simulink model "TVModel"  (R2022a)
settings: Solver=FixedStepDiscrete  StartTime=0.0  StopTime=10.0  FixedStep=0.02  MaxStep=0.01  RelTol=1e-3
undefined symbols (not defined in the file or in its folder): MB, TV, TV_OLD
libraries: simulink x22, simulink_extras x14, slpidlib x8, fuzblock x5, controlLib x4, dspstat3 x4, eeGeneralControl x3, cstblocks x3, eeSlidingModeController x1, sharedTrackingLibrary x1
(part 1 of 8)
settings Model: Creator=giuse  LastModifiedBy=Daniele
settings SolverCC: AutoInsertRateTranBlk=on
settings OptimizationCC: DefaultParameterBehavior=Inlined  UseDivisionForNetSlopeComputation=on  GainParamInheritBuiltInType=on  UseFloatMulNetSlope=on  InlineInvariantSignals=on  PassReuseOutputArgsAs=Individual arguments  ZeroExternalMemoryAtStartup=off  ZeroInternalMemoryAtStartup=off  NoFixptDivByZeroProtection=on  EfficientFloat2IntCast=on  LifeSpan=1  OptimizeBlockOrder=speed  DifferentSizesBufferReuse=on  EfficientTunableParamExpr=on
settings DebuggingCC: ParameterTunabilityLossMsg=error  UnconnectedInputMsg=warning  UnconnectedOutputMsg=warning  UnconnectedLineMsg=warning
settings HardwareCC: ProdBitPerPointer=32  ProdBitPerSizeT=32  ProdBitPerPtrDiffT=32  ProdLargestAtomicInteger=Long  ProdLargestAtomicFloat=Double  ProdWordSize=32  ProdLongLongMode=on  ProdHWDeviceType=ARM Compatible->ARM Cortex-M
settings SFSimCC: SimCustomHeaderCode="#include \"ITB_Nucleo_configuration\\Inc\\acados_wrapper.h\""  SimUserSources=ITB_Nucleo_configuration\Src\acados_wrapper.c  MATLABDynamicMemAlloc=off  CustomCodeUndefinedFunction=DoNotDetect
settings RTWCC: SystemTargetFile=ert.tlc  GenCodeOnly=on  TemplateMakefile=ert_default_tmf  RTWUseSimCustomCode=on  CustomHeaderCode="#include \"ITB_Nucleo_configuration\\Inc\\acados_wrapper.h\""  CustomSource=ITB_Nucleo_configuration\Src\acados_wrapper.c  DLArmComputeVersion=19.05
settings CodeAppCC: ForceParamTrailComments=on  IgnoreCustomStorageClasses=off  OperatorAnnotations=on  SimulinkDataObjDesc=on  SFDataObjDesc=on  CustomSymbolStrGlobalVar=rt$N$M  CustomSymbolStrType=$N$M  CustomSymbolStrFcn=$N$M$F  CustomSymbolStrMacro=$N$M  InsertBlockDesc=on
settings ERTTargetCC: TargetLangStandard=C99 (ISO)  GenerateSampleERTMain=on  IncludeMdlTerminateFcn=off  CombineOutputUpdateFcns=off  CombineSignalStateStructs=on  SupportAbsoluteTime=off  SupportComplex=off  SupportNonInlinedSFcns=on  InlinedParameterPlacement=NonHierarchical  ERTCustomFileTemplate=example_file_process.tlc  ERTFilePackagingFormat=CompactWithDataFile

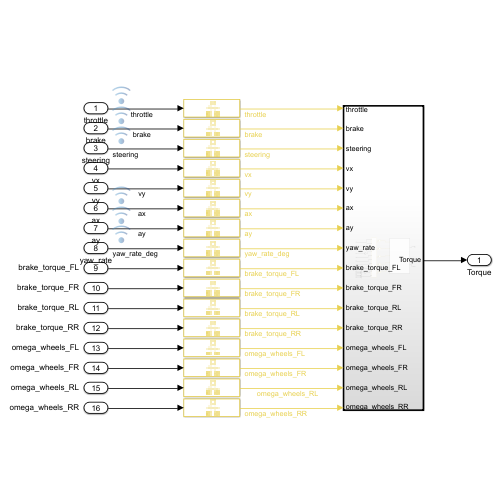
[thumbnail: Simulink's stored preview of the top-level diagram]
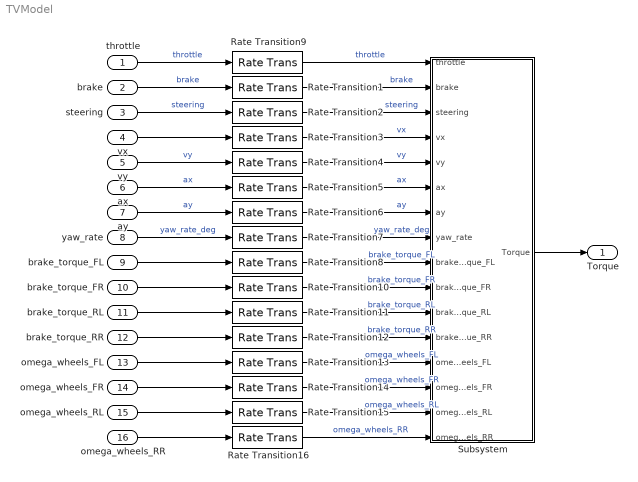
== system TVModel ==
  throttle : Inport  PortDimensions=1
  brake : Inport  Port=2  PortDimensions=1
  steering : Inport  Port=3  PortDimensions=1
  vx : Inport  Port=4  PortDimensions=1
  vy : Inport  Port=5  PortDimensions=1
  ax : Inport  Port=6  PortDimensions=1
  ay : Inport  Port=7  PortDimensions=1
  yaw_rate : Inport  Port=8  PortDimensions=1
  brake_torque_FL : Inport  Port=9  PortDimensions=1
  brake_torque_FR : Inport  Port=10  PortDimensions=1
  brake_torque_RL : Inport  Port=11  PortDimensions=1
  brake_torque_RR : Inport  Port=12  PortDimensions=1
  omega_wheels_FL : Inport  Port=13  PortDimensions=1
  omega_wheels_FR : Inport  Port=14  PortDimensions=1
  omega_wheels_RL : Inport  Port=15  PortDimensions=1
  omega_wheels_RR : Inport  Port=16  PortDimensions=1
  Rate Transition{1..16} (16 alike) : RateTransition  OutPortSampleTime=TV.MPC.T/TV.MPC.N
  Subsystem : Subsystem  TreatAsAtomicUnit=on  PartitionName=Subsystem
  Torque : Outport
  wires:
  vy/1 -> Rate Transition4/1  "vy"
  ax/1 -> Rate Transition5/1  "ax"
  brake/1 -> Rate Transition1/1  "brake"
  ay/1 -> Rate Transition6/1  "ay"
  brake_torque_RL/1 -> Rate Transition11/1
  brake_torque_RR/1 -> Rate Transition12/1
  omega_wheels_RR/1 -> Rate Transition16/1
  omega_wheels_FL/1 -> Rate Transition13/1
  brake_torque_FR/1 -> Rate Transition10/1
  yaw_rate/1 -> Rate Transition7/1  "yaw_rate_deg"
  omega_wheels_FR/1 -> Rate Transition14/1
  omega_wheels_RL/1 -> Rate Transition15/1
  steering/1 -> Rate Transition2/1  "steering"
  brake_torque_FL/1 -> Rate Transition8/1
  vx/1 -> Rate Transition3/1
  throttle/1 -> Rate Transition9/1  "throttle"
  Subsystem/1(Torque) -> Torque/1
  Rate Transition9/1 -> Subsystem/1(throttle)  "throttle"
  Rate Transition1/1 -> Subsystem/2(brake)  "brake"
  Rate Transition2/1 -> Subsystem/3(steering)  "steering"
  Rate Transition3/1 -> Subsystem/4(vx)  "vx"
  Rate Transition4/1 -> Subsystem/5(vy)  "vy"
  Rate Transition5/1 -> Subsystem/6(ax)  "ax"
  Rate Transition6/1 -> Subsystem/7(ay)  "ay"
  Rate Transition7/1 -> Subsystem/8(yaw_rate)  "yaw_rate_deg"
  Rate Transition8/1 -> Subsystem/9(brake_torque_FL)  "brake_torque_FL"
  Rate Transition10/1 -> Subsystem/10(brake_torque_FR)  "brake_torque_FR"
  Rate Transition11/1 -> Subsystem/11(brake_torque_RL)  "brake_torque_RL"
  Rate Transition12/1 -> Subsystem/12(brake_torque_RR)  "brake_torque_RR"
  Rate Transition13/1 -> Subsystem/13(omega_wheels_FL)  "omega_wheels_FL"
  Rate Transition14/1 -> Subsystem/14(omega_wheels_FR)  "omega_wheels_FR"
  Rate Transition15/1 -> Subsystem/15(omega_wheels_RL)  "omega_wheels_RL"
  Rate Transition16/1 -> Subsystem/16(omega_wheels_RR)  "omega_wheels_RR"

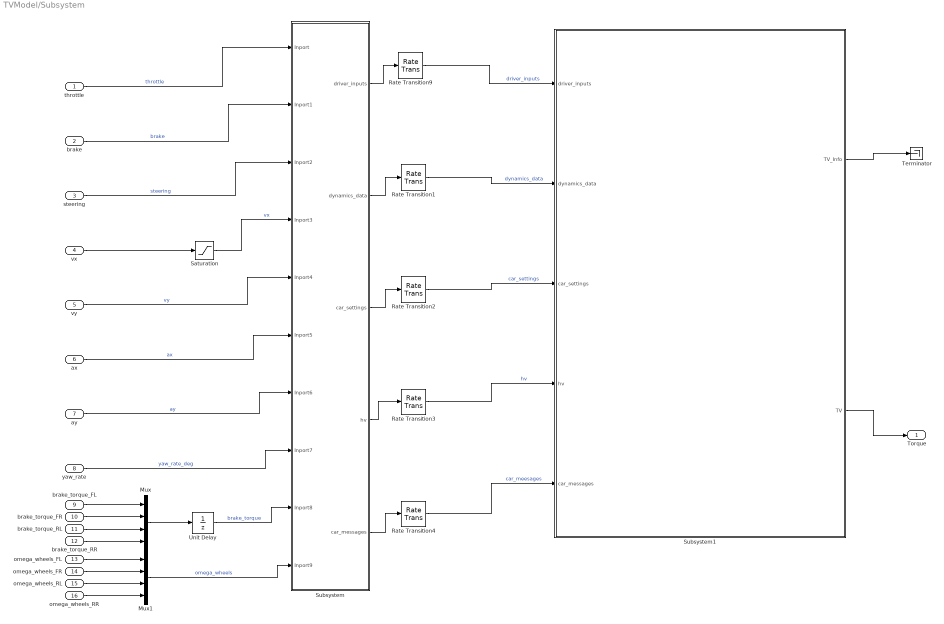
== system TVModel/Subsystem ==
  throttle : Inport  SampleTime=0.02
  brake : Inport  Port=2
  steering : Inport  Port=3
  vx : Inport  Port=4
  vy : Inport  Port=5
  ax : Inport  Port=6
  ay : Inport  Port=7
  yaw_rate : Inport  Port=8
  brake_torque_FL : Inport  Port=9
  brake_torque_FR : Inport  Port=10
  brake_torque_RL : Inport  Port=11
  brake_torque_RR : Inport  Port=12
  omega_wheels_FL : Inport  Port=13
  omega_wheels_FR : Inport  Port=14
  omega_wheels_RL : Inport  Port=15
  omega_wheels_RR : Inport  Port=16
  Mux : Mux
  Mux1 : Mux
  Rate Transition{1..4,9} (5 alike) : RateTransition  OutPortSampleTime=TV.MPC.T/TV.MPC.N
  Saturation : Saturate  UpperLimit=inf  LowerLimit=0
  Subsystem : Subsystem
  Subsystem1 : Subsystem
  Terminator : Terminator
  Unit Delay : UnitDelay  SampleTime=-1  HasFrameUpgradeWarning=on
  Torque : Outport
  wires:
  omega_wheels_FL/1 -> Mux1/1
  ax/1 -> Subsystem/6(Inport5)  "ax"
  Unit Delay/1 -> Subsystem/9(Inport8)  "brake_torque"
  vy/1 -> Subsystem/5(Inport4)  "vy"
  ay/1 -> Subsystem/7(Inport6)  "ay"
  Mux1/1 -> Subsystem/10(Inport9)  "omega_wheels"
  Saturation/1 -> Subsystem/4(Inport3)  "vx"
  brake/1 -> Subsystem/2(Inport1)  "brake"
  yaw_rate/1 -> Subsystem/8(Inport7)  "yaw_rate_deg"
  throttle/1 -> Subsystem/1(Inport)  "throttle"
  brake_torque_RL/1 -> Mux/3
  vx/1 -> Saturation/1
  brake_torque_FL/1 -> Mux/1
  omega_wheels_RR/1 -> Mux1/4
  brake_torque_RR/1 -> Mux/4
  steering/1 -> Subsystem/3(Inport2)  "steering"
  omega_wheels_FR/1 -> Mux1/2
  Mux/1 -> Unit Delay/1
  omega_wheels_RL/1 -> Mux1/3
  brake_torque_FR/1 -> Mux/2
  Subsystem/1(driver_inputs) -> Rate Transition9/1
  Subsystem/2(dynamics_data) -> Rate Transition1/1
  Subsystem/5(car_messages) -> Rate Transition4/1
  Subsystem/3(car_settings) -> Rate Transition2/1
  Rate Transition4/1 -> Subsystem1/5(car_messages)  "car_meesages"
  Rate Transition3/1 -> Subsystem1/4(hv)  "hv"
  Rate Transition2/1 -> Subsystem1/3(car_settings)  "car_settings"
  Rate Transition1/1 -> Subsystem1/2(dynamics_data)  "dynamics_data"
  Subsystem1/2(TV) -> Torque/1
  Subsystem1/1(TV_Info) -> Terminator/1
  Rate Transition9/1 -> Subsystem1/1(driver_inputs)  "driver_inputs"
  Subsystem/4(hv) -> Rate Transition3/1

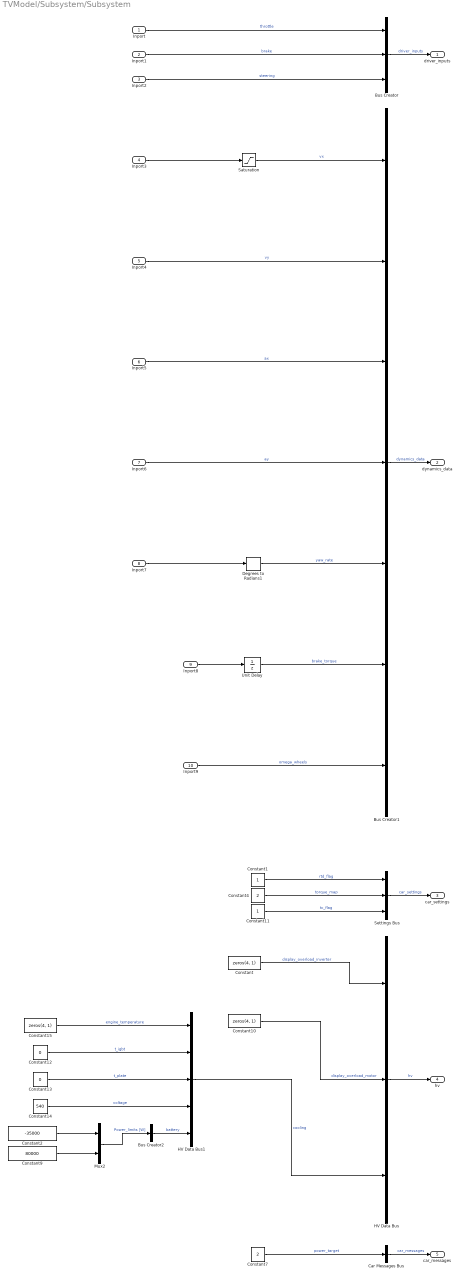
== system TVModel/Subsystem/Subsystem ==
  Inport : Inport
  Inport1 : Inport  Port=2
  Inport2 : Inport  Port=3
  Inport3 : Inport  Port=4
  Inport4 : Inport  Port=5
  Inport5 : Inport  Port=6
  Inport6 : Inport  Port=7
  Inport7 : Inport  Port=8
  Inport8 : Inport  Port=9
  Inport9 : Inport  Port=10
  Bus Creator : BusCreator  Inputs=3
  Bus Creator1 : BusCreator  Inputs=7
  Bus Creator2 : BusCreator  Inputs=1
  Car Messages Bus : BusCreator  Inputs=1
  Constant : Constant  Value=zeros(4, 1)
  Constant1 : Constant  OutDataTypeStr=uint8
  Constant10 : Constant  Value=zeros(4, 1)
  Constant11 : Constant  OutDataTypeStr=uint8
  Constant12 : Constant  Value=0
  Constant13 : Constant  Value=0
  Constant14 : Constant  Value=540
  Constant15 : Constant  Value=zeros(4, 1)
  Constant2 : Constant  Value=-35000
  Constant4 : Constant  Value=2  OutDataTypeStr=uint8
  Constant7 : Constant  Value=2
  Constant9 : Constant  Value=80000
  Degrees to Radians1 : simulink_extras/Transformations/Degrees to Radians
  HV Data Bus : BusCreator  Inputs=3
  HV Data Bus1 : BusCreator  Inputs=5
  Mux2 : Mux  Inputs=2
  Saturation : Saturate  UpperLimit=inf  LowerLimit=0
  Settings Bus : BusCreator  Inputs=3
  Unit Delay : UnitDelay  SampleTime=-1  HasFrameUpgradeWarning=on
  driver_inputs : Outport
  dynamics_data : Outport  Port=2
  car_settings : Outport  Port=3
  hv : Outport  Port=4
  car_messages : Outport  Port=5
  wires:
  Constant4/1 -> Settings Bus/2  "torque_map"
  Inport2/1 -> Bus Creator/3  "steering"
  Constant1/1 -> Settings Bus/1  "rtd_flag"
  Car Messages Bus/1 -> car_messages/1  "car_messages"
  Inport9/1 -> Bus Creator1/7  "omega_wheels"
  Degrees to Radians1/1 -> Bus Creator1/5  "yaw_rate"
  Constant7/1 -> Car Messages Bus/1  "power_target"
  Bus Creator/1 -> driver_inputs/1  "driver_inputs"
  Inport7/1 -> Degrees to Radians1/1
  Settings Bus/1 -> car_settings/1  "car_settings"
  Bus Creator1/1 -> dynamics_data/1  "dynamics_data"
  Constant11/1 -> Settings Bus/3  "tc_flag"
  Inport6/1 -> Bus Creator1/4  "ay"
  Inport5/1 -> Bus Creator1/3  "ax"
  Inport4/1 -> Bus Creator1/2  "vy"
  Inport/1 -> Bus Creator/1  "throttle"
  Unit Delay/1 -> Bus Creator1/6  "brake_torque"
  Inport8/1 -> Unit Delay/1
  Inport1/1 -> Bus Creator/2  "brake"
  Saturation/1 -> Bus Creator1/1  "vx"
  Inport3/1 -> Saturation/1
  HV Data Bus/1 -> hv/1  "hv"
  Mux2/1 -> Bus Creator2/1  "Power_limits [W]"
  Constant10/1 -> HV Data Bus/2  "display_overload_motor"
  HV Data Bus1/1 -> HV Data Bus/3  "cooling"
  Constant/1 -> HV Data Bus/1  "display_overload_inverter"
  Constant14/1 -> HV Data Bus1/4  "voltage"
  Constant12/1 -> HV Data Bus1/2  "t_igbt"
  Constant2/1 -> Mux2/1
  Constant13/1 -> HV Data Bus1/3  "t_plate"
  Constant9/1 -> Mux2/2
  Bus Creator2/1 -> HV Data Bus1/5  "battery"
  Constant15/1 -> HV Data Bus1/1  "engine_temperature"

== system TVModel/Subsystem/Subsystem1 ==
  In Bus Element2 : Inport  PortName=driver_inputs
  In Bus Element5 : Inport  PortName=driver_inputs
  In Bus Element11 : Inport  PortName=driver_inputs
  In Bus Element3 : Inport  Port=2  PortName=dynamics_data
  In Bus Element4 : Inport  Port=2  PortName=dynamics_data
  In Bus Element8 : Inport  Port=2  PortName=dynamics_data
  In Bus Element6 : Inport  Port=3  PortName=car_settings
  In Bus Element10 : Inport  Port=3  PortName=car_settings
  In Bus Element1 : Inport  Port=3  PortName=car_settings
  In Bus Element7 : Inport  Port=4  PortName=hv
  In Bus Element9 : Inport  Port=4  PortName=hv
  In Bus Element : Inport  Port=5  PortName=car_messages
  Data Store_General_Params : DataStoreMemory  DataStoreName=General_Params  WriteAfterWriteMsg=warning  WriteAfterReadMsg=warning  InitialValue=TV.LV.GENERAL  ShowAdditionalParam=off  OutDataTypeStr=Bus: zGeneral_Params
  Data Store_Map_Params : DataStoreMemory  DataStoreName=Map_Params  WriteAfterWriteMsg=warning  WriteAfterReadMsg=warning  InitialValue=TV.LV.MAP  ShowAdditionalParam=off  OutDataTypeStr=Bus: zMap_Params
  Slip Control : Subsystem
      settings: PortSchema="{\"entries\":[{\"content\":{\"sides\":[{\"content\":{\"connectorIds\":[\"In1\",\"In2\",\"In3\",\"In4\",\"In5\",\"In6\"]},\"type\":\"ConnectorPlacement.EquallySpacedRectSide\",\"uuid\":\"0a8dcb05-2d5e-427e-b3e7-e0a9c36078aa\"},{\"content\":{\"connectorIds\":[\"Out1\",\"Out2\"],\"side\":\"RIGHT\"},\"type\":\"ConnectorPlacement.EquallySpacedRectSide\",\"uuid\":\"4a483d6b-4a8b-4193-8822-91ed85f9d11c\"},{\"content\":{\"connectorIds\":[\"Out3\"],\"side\":\"TOP\"},\"type\":\"ConnectorPlacement.EquallySpacedRectSide\",\"uuid\":\"653aa866-b257-425a-9060-0af71437e8f6\"}]},\"type\":\"ConnectorPlacement.EquallySpacedConnector\",\"uuid\":\"85fc9358-bdaa-4ddd-978c-a41ea6d8fd7a\"}],\"packageUris\":[\"http://schema.mathworks.com/mf0/Connector/R2020b\"],\"version\":\"1.0\"}"
      mask Display: image('$imagefile'); % Use "Edit Image" on toolstrip to change.
  Terminator : Terminator
  Torque Distribution : Subsystem
      settings: PortSchema="{\"entries\":[{\"content\":{\"sides\":[{\"content\":{\"connectorIds\":[\"In1\",\"In2\",\"In3\",\"In4\",\"In5\",\"In6\",\"In7\",\"In8\",\"Out3\",\"In9\"]},\"type\":\"ConnectorPlacement.EquallySpacedRectSide\",\"uuid\":\"ece1a4aa-f225-4de9-8190-960458904133\"},{\"content\":{\"connectorIds\":[\"Out1\",\"Out2\"],\"side\":\"RIGHT\"},\"type\":\"ConnectorPlacement.EquallySpacedRectSide\",\"uuid\":\"588db727-2c2c-47b1-ab80-0176258858bf\"},{\"content\":{\"connectorIds\":[],\"side\":\"TOP\"},\"type\":\"ConnectorPlacement.EquallySpacedRectSide\",\"uuid\":\"54ce6245-2304-4750-b056-247655cbbdc1\"}]},\"type\":\"ConnectorPlacement.EquallySpacedConnector\",\"uuid\":\"9c8e646c-fa54-49ed-932c-87ddbb4d1884\"}],\"packageUris\":[\"http://schema.mathworks.com/mf0/Connector/R2020b\"],\"version\":\"1.0\"}"
      mask Display: image('$imagefile'); % Use "Edit Image" on toolstrip to change.
  Torque Limits : Subsystem
      mask Display: image('$imagefile'); % Use "Edit Image" on toolstrip to change.
  regen_brake : Subsystem
  steering_to_front_wheels : Subsystem
  Out Bus Element4 : Outport  PortName=TV_Info  Element=Torque_Distribution
  Out Bus Element6 : Outport  PortName=TV_Info  Element=Input_Signals.hv
  Out Bus Element7 : Outport  PortName=TV_Info  Element=Input_Signals.car_settings
  Out Bus Element8 : Outport  PortName=TV_Info  Element=Input_Signals.dynamics_data
  Out Bus Element9 : Outport  PortName=TV_Info  Element=Input_Signals.driver_inputs
  Out Bus Element10 : Outport  PortName=TV_Info  Element=Slip_Control
  Out Bus Element : Outport  Port=2  PortName=TV
  wires:
  regen_brake/1(brake_signal) -> Torque Distribution/3(brake_signal)
  In Bus Element8/1 -> Torque Limits/2(dynamics_data), Out Bus Element8/1  "dynamics_data"
  In Bus Element10/1 -> Torque Distribution/7(Car_Settings)
  In Bus Element2/1 -> steering_to_front_wheels/1(driver_inputs), regen_brake/1(driver_inputs), Torque Distribution/2(driver_inputs)
  steering_to_front_wheels/1(front_wheels_steering) -> Torque Distribution/4(front_wheels_steering), Slip Control/1(front_wheels_steering)
  In Bus Element3/1 -> Torque Distribution/1(dynamics_data)
  In Bus Element4/1 -> Slip Control/2(dynamics_data)
  Slip Control/2(slip_ratio) -> Torque Distribution/6(slip_ratio)
  Torque Distribution/1(TV_info) -> Out Bus Element4/1
  Torque Limits/1(torque_limits) -> Torque Distribution/9(torque_limits), Slip Control/4(torque_limits)
  Torque Distribution/2(TV) -> Out Bus Element/1
  Torque Distribution/3(TC_torque_out) -> Slip Control/5(tv)
  Slip Control/3(TV_Info) -> Out Bus Element10/1
  In Bus Element7/1 -> Out Bus Element6/1, Torque Limits/4(hv)
  In Bus Element11/1 -> Slip Control/6(driver_inputs)
  In Bus Element9/1 -> Torque Distribution/8(hv)
  In Bus Element5/1 -> Torque Limits/1(driver_inputs), Out Bus Element9/1  "driver_inputs"
  In Bus Element1/1 -> Slip Control/3(car_settings)
  Slip Control/1(TC_Torque) -> Torque Distribution/5(TC_Torque)
  In Bus Element6/1 -> Out Bus Element7/1, Torque Limits/3(car_settings)  "car_settings"
  In Bus Element/1 -> Terminator/1

== system TVModel/Subsystem/Subsystem1/Slip Control ==
  In Bus Element6 : Inport  PortName=front_wheels_steering
  In Bus Element5 : Inport  PortName=front_wheels_steering
  In Bus Element1 : Inport  Port=2  PortName=dynamics_data
  In Bus Element3 : Inport  Port=2  PortName=dynamics_data
  In Bus Element2 : Inport  Port=3  PortName=car_settings
  In Bus Element : Inport  Port=4  PortName=torque_limits
  In Bus Element7 : Inport  Port=5  PortName=tv
  In Bus Element4 : Inport  Port=6  PortName=driver_inputs
  Slip Ratios : Subsystem
  Traction Control : Subsystem
  Out Bus Element1 : Outport  PortName=TC_Torque
  Out Bus Element : Outport  Port=2  PortName=slip_ratio
  Out Bus Element7 : Outport  Port=3  PortName=TV_Info  Element=Slip_Ratios
  wires:
  Slip Ratios/1(slip_ratio) -> Traction Control/5(slip_ratio), Out Bus Element/1  "slip_ratio"
  In Bus Element1/1 -> Slip Ratios/1(dynamics_data)  "dynamics_data"
  In Bus Element6/1 -> Slip Ratios/2(front_wheels_steering)
  Slip Ratios/2(TV_Info) -> Out Bus Element7/1
  Traction Control/1(TC_Torque) -> Out Bus Element1/1
  In Bus Element2/1 -> Traction Control/2(car_settings)
  In Bus Element/1 -> Traction Control/3(torque_limits)
  In Bus Element7/1 -> Traction Control/1(tv)
  In Bus Element3/1 -> Traction Control/4(dynamics_data)
  In Bus Element4/1 -> Traction Control/6(driver_inputs)
  In Bus Element5/1 -> Traction Control/7(front_wheels_steering)

== system TVModel/Subsystem/Subsystem1/Torque Distribution ==
  In Bus Element : Inport  PortName=dynamics_data
  In Bus Element1 : Inport  Port=2  PortName=driver_inputs
  In Bus Element9 : Inport  Port=2  PortName=driver_inputs
  In Bus Element3 : Inport  Port=3  PortName=brake_signal
  In Bus Element2 : Inport  Port=4  PortName=front_wheels_steering
  In Bus Element6 : Inport  Port=4  PortName=front_wheels_steering
  In Bus Element7 : Inport  Port=5  PortName=TC_Torque
  In Bus Element5 : Inport  Port=6  PortName=slip_ratio
  In Bus torque_map : Inport  Port=7  PortName=Car_Settings
  In Bus Element8 : Inport  Port=8  PortName=hv
  In Bus Element4 : Inport  Port=9  PortName=torque_limits
  MPC : Subsystem
      mask Display: image('$imagefile'); % Use "Edit Image" on toolstrip to change.
  Reference Tracking : Subsystem
      settings: PortSchema="{\"entries\":[{\"content\":{\"sides\":[{\"content\":{\"connectorIds\":[\"In1\",\"In2\",\"In3\"]},\"type\":\"ConnectorPlacement.EquallySpacedRectSide\",\"uuid\":\"f6b455b0-1993-4661-a7e5-67ec12298593\"},{\"content\":{\"connectorIds\":[\"Out1\"],\"side\":\"RIGHT\"},\"type\":\"ConnectorPlacement.EquallySpacedRectSide\",\"uuid\":\"cda4fcfc-381a-4065-8f38-4c677ea159cd\"},{\"content\":{\"connectorIds\":[\"Out2\"],\"side\":\"TOP\"},\"type\":\"ConnectorPlacement.EquallySpacedRectSide\",\"uuid\":\"ea61d581-e491-4d68-abf5-6728fc8d29b2\"}]},\"type\":\"ConnectorPlacement.EquallySpacedConnector\",\"uuid\":\"4f7fa02a-c913-4d0a-a26f-e6c9629c03da\"}],\"packageUris\":[\"http://schema.mathworks.com/mf0/Connector/R2020b\"],\"version\":\"1.0\"}"
      mask Display: image('$imagefile'); % Use "Edit Image" on toolstrip to change.
  Out Bus Element1 : Outport  PortName=TV_info  Element=MPC
  Out Bus Element : Outport  PortName=TV_info  Element=Reference
  Out Bus Element18 : Outport  Port=2  PortName=TV
  Out Bus Element2 : Outport  Port=3  PortName=TC_torque_out
  wires:
  In Bus torque_map/1 -> MPC/9(Car_Setting)
  In Bus Element5/1 -> MPC/4(slip_ratio)
  In Bus Element4/1 -> MPC/1(torque_limits)  "torque_limits_signals"
  In Bus Element3/1 -> MPC/7(brake_signal)  "regen"
  In Bus Element2/1 -> MPC/6(front_wheel_angles)  "front_wheels_steering_signals"
  Reference Tracking/1(yaw_rate_desired) -> MPC/3(yaw_rate_desired)  "yaw_rate_desired"
  In Bus Element/1 -> Reference Tracking/1(dynamics_data), MPC/2(dynamics_data)
  In Bus Element1/1 -> MPC/5(driver_inputs)  "driver_inputs_signals"
  In Bus Element6/1 -> Reference Tracking/2(front_wheels_steering)
  Reference Tracking/2(TV_Info) -> Out Bus Element/1
  MPC/1(TV_Info) -> Out Bus Element1/1
  In Bus Element7/1 -> MPC/8(TC_Torque)
  In Bus Element8/1 -> MPC/10(hv)  "hv"
  MPC/2(TV) -> Out Bus Element18/1
  MPC/3(TC_torque_out) -> Out Bus Element2/1
  In Bus Element9/1 -> Reference Tracking/3(driver_inputs)  "driver_inputs_signals"

== system TVModel/Subsystem/Subsystem1/Torque Limits ==
  In Bus throttle : Inport  PortName=driver_inputs
  In Bus Element6 : Inport  Port=2  PortName=dynamics_data
  In Bus Element3 : Inport  Port=2  PortName=dynamics_data
  In Bus torque_map1 : Inport  Port=3  PortName=car_settings
  In Bus torque_map3 : Inport  Port=3  PortName=car_settings
  In Bus torque_map2 : Inport  Port=3  PortName=car_settings
  In Bus Element2 : Inport  Port=4  PortName=hv
  In Bus Element1 : Inport  Port=4  PortName=hv
  Torque Limits Positive : Subsystem
  Torque Limits Regen : Subsystem
  Torque Request : Subsystem
  Out Bus Element : Outport  PortName=torque_limits  Element=t_req
  Out Bus Element2 : Outport  PortName=torque_limits  Element=t_limit_positive
  Out Bus Element4 : Outport  PortName=torque_limits  Element=t_limit_negative
  wires:
  Torque Limits Regen/1(t_limit_regen) -> Out Bus Element4/1  "t_limit_negative"
  Torque Limits Positive/1(t_limit_positive) -> Out Bus Element2/1  "t_limit_positive"
  Torque Request/1(t_req) -> Out Bus Element/1  "t_req"
  In Bus throttle/1 -> Torque Request/1(driver_inputs)  "throttle"
  In Bus torque_map3/1 -> Torque Request/2(Car_Settings)  "torque_map"
  In Bus Element2/1 -> Torque Limits Positive/2(hv)  "hv"
  In Bus Element6/1 -> Torque Limits Positive/3(dynamics_data)  "omega_wheels"
  In Bus torque_map1/1 -> Torque Limits Positive/1(car_settings)  "torque_map"
  In Bus torque_map2/1 -> Torque Limits Regen/1(car_settings)  "torque_map"
  In Bus Element1/1 -> Torque Limits Regen/2(hv)  "hv"
  In Bus Element3/1 -> Torque Limits Regen/3(dynamics_data)  "omega_wheels"

== system TVModel/Subsystem/Subsystem1/regen_brake ==
  In Bus Element : Inport  PortName=driver_inputs  Element=brake
  Gain : Gain  Gain=1/0.28
  Saturation : Saturate  UpperLimit=1  LowerLimit=0
  Out Bus Element : Outport  PortName=brake_signal  Element=regen
  wires:
  Gain/1 -> Saturation/1
  In Bus Element/1 -> Gain/1
  Saturation/1 -> Out Bus Element/1

== system TVModel/Subsystem/Subsystem1/steering_to_front_wheels ==
  In Bus Element : Inport  PortName=driver_inputs  Element=steering
  In Bus Element1 : Inport  PortName=driver_inputs  Element=steering
  Abs : Abs  SaturateOnIntegerOverflow=off
  Divide1 : Product  Inputs=**
  Mux : Mux  Inputs=2
  Sign : Signum
  Unary Minus : UnaryMinus
  steering_to_wheel_angle_single_axis_LUT : Lookup_n-D  NumberOfTableDimensions=1  BreakpointsForDimension1=TV.LUT.Car_LUT.steer_at_ground_single_axis_LUT.Steering  Table=TV.LUT.Car_LUT.steer_at_ground_single_axis_LUT.SteerAngle_SingleAxis  InternalRulePriority=Speed  RndMeth=Simplest
  steering_to_wheel_angles_LUT : Lookup_n-D  NumberOfTableDimensions=1  BreakpointsForDimension1=TV.LUT.Car_LUT.steer_at_ground_LUT.Steering  Table=TV.LUT.Car_LUT.steer_at_ground_LUT.SteerAngle_FL  InternalRulePriority=Speed  RndMeth=Simplest
  Out Bus Element : Outport  PortName=front_wheels_steering  Element=single_axis
  Out Bus Element1 : Outport  PortName=front_wheels_steering  Element=different_axis
  wires:
  Divide1/1 -> Out Bus Element1/1  "front_wheel_angle_single_axis_different_axis"
  steering_to_wheel_angle_single_axis_LUT/1 -> Out Bus Element/1  "front_wheel_angle_single_axis"
  Sign/1 -> Divide1/2
  Unary Minus/1 -> Mux/2
  In Bus Element/1 -> steering_to_wheel_angle_single_axis_LUT/1
  steering_to_wheel_angles_LUT/1 -> Abs/1  "front_wheel_angles"
  Mux/1 -> steering_to_wheel_angles_LUT/1
  Abs/1 -> Divide1/1
  In Bus Element1/1 -> Sign/1, Mux/1, Unary Minus/1

== system TVModel/Subsystem/Subsystem1/Slip Control/Slip Ratios ==
  In Bus Element{,2,4..5} (4 alike) : Inport  PortName=dynamics_data
  In Bus Element6 : Inport  Port=2  PortName=front_wheels_steering
  In Bus Element1 : Inport  Port=2  PortName=front_wheels_steering
  FL SR : Subsystem
  FR SR : Subsystem
  "RL RR " : Subsystem
  RL SR : Subsystem
  Out Bus Element : Outport  PortName=slip_ratio  Element=fl
  Out Bus Element1 : Outport  PortName=slip_ratio  Element=fr
  Out Bus Element2 : Outport  PortName=slip_ratio  Element=rl
  Out Bus Element3 : Outport  PortName=slip_ratio  Element=rr
  Out Bus Element4 : Outport  Port=2  PortName=TV_Info  Element=slip_ratio_fl
  Out Bus Element5 : Outport  Port=2  PortName=TV_Info  Element=slip_ratio_fr
  Out Bus Element6 : Outport  Port=2  PortName=TV_Info  Element=slip_ratio_rl
  Out Bus Element7 : Outport  Port=2  PortName=TV_Info  Element=slip_ratio_rr
  wires:
  In Bus Element5/1 -> "RL RR "/1(dynamics_data)
  In Bus Element4/1 -> RL SR/1(dynamics_data)
  In Bus Element2/1 -> FR SR/1(dynamics_data)
  In Bus Element1/1 -> FR SR/2(front_wheels_steering)
  In Bus Element6/1 -> FL SR/2(front_wheels_steering)
  In Bus Element/1 -> FL SR/1(dynamics_data)
  "RL RR "/1(RR) -> Out Bus Element7/1, Out Bus Element3/1  "kappa_RR"
  FR SR/1(FR) -> Out Bus Element5/1, Out Bus Element1/1  "kappa_FR"
  FL SR/1(FL) -> Out Bus Element4/1, Out Bus Element/1  "kappa_FL"
  RL SR/1(RL) -> Out Bus Element6/1, Out Bus Element2/1  "kappa_RL"

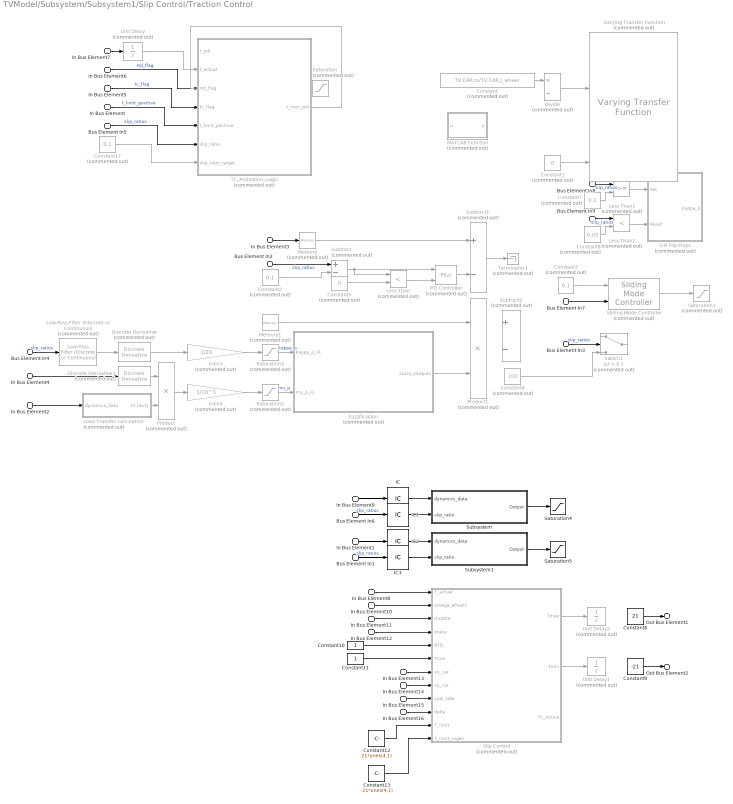
== system TVModel/Subsystem/Subsystem1/Slip Control/Traction Control ==
  In Bus Element7 : Inport  PortName=tv
  In Bus Element3 : Inport  PortName=tv
  In Bus Element8 : Inport  PortName=tv
  In Bus Element6 : Inport  Port=2  PortName=car_settings  Element=rtd_flag
  In Bus Element5 : Inport  Port=2  PortName=car_settings  Element=tc_flag
  In Bus Element : Inport  Port=3  PortName=torque_limits  Element=t_limit_positive
  In Bus Element2 : Inport  Port=4  PortName=dynamics_data
  In Bus Element9 : Inport  Port=4  PortName=dynamics_data
  In Bus Element1 : Inport  Port=4  PortName=dynamics_data
  In Bus Element4 : Inport  Port=4  PortName=dynamics_data  Element=ax
  In Bus Element10 : Inport  Port=4  PortName=dynamics_data  Element=omega_wheels
  In Bus Element13 : Inport  Port=4  PortName=dynamics_data  Element=vx
  In Bus Element14 : Inport  Port=4  PortName=dynamics_data  Element=vy
  In Bus Element15 : Inport  Port=4  PortName=dynamics_data  Element=yaw_rate
  Bus Element In{1..9} (9 alike) : Inport  Port=5  PortName=slip_ratio
  In Bus Element11 : Inport  Port=6  PortName=driver_inputs  Element=throttle
  In Bus Element12 : Inport  Port=6  PortName=driver_inputs  Element=brake
  In Bus Element16 : Inport  Port=7  PortName=front_wheels_steering  Element=single_axis
  Constant : Constant  Commented=on  Value=TV.CAR.rs/TV.CAR.J_wheel
  Constant1 : Constant  Commented=on  Value=0
  Constant10 : Constant
  Constant11 : Constant
  Constant12 : Constant  Value=21*ones(4,1)
  Constant13 : Constant  Value=-21*ones(4,1)
  Constant{2..3,7,17} (4 alike) : Constant  Commented=on  Value=0.1
  Constant4 : Constant  Commented=on  Value=100
  Constant5 : Constant  Commented=on  Value=0
  Constant6 : Constant  Value=21
  Constant8 : Constant  Commented=on  Value=0.05
  Constant9 : Constant  Value=-21
  Discrete Derivative : simulink/Discrete/Discrete Derivative  Commented=on  gainval=1.0  ICPrevScaledInput=0.0  OutMin=[]  OutMax=[]  OutDataType=fixdt(1, 16)  OutScaling=2^-10  DoSatur=off
  Discrete Derivative1 : simulink/Discrete/Discrete Derivative  Commented=on  gainval=1.0  ICPrevScaledInput=0.0  OutMin=[]  OutMax=[]  OutDataType=fixdt(1, 16)  OutScaling=2^-10  DoSatur=off
  Divide : Product  Commented=on  Inputs=*/
  Fuzzification : Subsystem  Commented=on
  Gain3 : Gain  Commented=on  Gain=1/20
  Gain4 : Gain  Commented=on  Gain=1/10^3
  IC{,1..3} (4 alike) : InitialCondition  Value=0
  Less Than : RelationalOperator  Commented=on  Operator=<  OutDataTypeStr=boolean  RndMeth=Simplest  InputSameDT=off
  Less Than1 : RelationalOperator  Commented=on  OutDataTypeStr=boolean  RndMeth=Simplest  InputSameDT=off
  Less Than2 : RelationalOperator  Commented=on  Operator=<  OutDataTypeStr=boolean  RndMeth=Simplest  InputSameDT=off
  Load Transfer calculation : Subsystem  Commented=on
  Low-Pass Filter (Discrete or Continuous) : eeGeneralControl/Low-Pass Filter (Discrete or Continuous)  Commented=on  K=1  T=1/(2*pi*3)  B=inf  A=-inf  init_option=Inherited from block input  x0=0  Ts=-1
  MATLAB Function : MATLAB Function  Commented=on  TreatAsAtomicUnit=on
  Memory : Memory  Commented=on  InheritSampleTime=on
  Memory1 : Memory  Commented=on  InheritSampleTime=on
  PID Controller : slpidlib/PID Controller  Commented=on  Controller=PI  Form=Parallel  TimeDomain=Discrete-time  UseExternalTs=off  SampleTime=-1  IntegratorMethod=Forward Euler  FilterMethod=Forward Euler  ControllerParametersSource=internal  P=2  I=5  UseKiTs=off  D=0  N=100  UseFilter=on  TunerSelectOption=Transfer Function Based (PID Tuner App)  InitialConditionSource=internal  InitialConditionForIntegrator=0  InitialConditionForFilter=0  DifferentiatorICPrevScaledInput=0  ExternalReset=level  TrackingMode=off  Kt=1  LimitOutput=off  SatLimitsSource=internal  UpperSaturationLimit=inf  LowerSaturationLimit=-inf  LinearizeAsGain=on  AntiWindupMode=none  Kb=1  POutMin=[]  POutMax=[]  IOutMin=[]  IOutMax=[]  DOutMin=[]  DOutMax=[]  NOutMin=[]  NOutMax=[]  SumOutMin=[]  SumOutMax=[]  SaturationOutMin=[]  SaturationOutMax=[]  PParamMin=[]  PParamMax=[]  IParamMin=[]  IParamMax=[]  DParamMin=[]  DParamMax=[]  NParamMin=[]  NParamMax=[]  KbParamMin=[]  KbParamMax=[]  KtParamMin=[]  KtParamMax=[]  KbOutMin=[]  KbOutMax=[]  KtOutMin=[]  KtOutMax=[]  IntegratorOutMin=[]  IntegratorOutMax=[]  FilterOutMin=[]  FilterOutMax=[]  SumI1OutMin=[]  SumI1OutMax=[]  SumI2OutMin=[]  SumI2OutMax=[]  SumI3OutMin=[]  SumI3OutMax=[]  SumI4OutMin=[]  SumI4OutMax=[]  SumDOutMin=[]  SumDOutMax=[]  DifferentiatorOutMin=[]  DifferentiatorOutMax=[]  FilterDiffOutCoefMin=[]  FilterDiffOutCoefMax=[]  ReciprocalOutMin=[]  ReciprocalOutMax=[]  SumDenOutMin=[]  SumDenOutMax=[]  SumNumOutMin=[]  SumNumOutMax=[]  DivideOutMin=[]  DivideOutMax=[]  UdiffTsProdOutMin=[]  UdiffTsProdOutMax=[]  NTsProdOutMin=[]  NTsProdOutMax=[]  UintegralTsProdOutMin=[]  UintegralTsProdOutMax=[]  UngainTsProdOutMin=[]  UngainTsProdOutMax=[]  IntegratorContinuousStateAttributes=''  IntegratorStateMustResolveToSignalObject=off  IntegratorRTWStateStorageClass=Auto  FilterContinuousStateAttributes=''  FilterStateMustResolveToSignalObject=off  FilterRTWStateStorageClass=Auto  ParallelPVariant=InternalParameters  IdealPVariant=Disabled  IVariant=InternalParameters  DVariant=Disabled  IntegratorVariant=Discrete  SatVariant=Disabled  AWVariant=Passthrough  PCopyVariant=Disabled  TRVariant=Disabled  FdbkBlocksVariant=Forward  IdealPFdbkVariant=Disabled  SatFdbkVariant=Disabled  DerivativeFilterVariant=Disabled  NVariant=Disabled  NCopyVariant=Disabled_SignalSpec  FilterICVariant=Disabled  IntegratorICVariant=InternalICs  ExternalResetVariant=ExternalReset  TRSumVariant=Passthrough  SumFdbkVariant=Disabled  SumVariant=Sum_PI  TsampFilterVariant=InternalTs  TsampNgainVariant=Passthrough  TsampIntegralVariant=Passthrough  ExternalSaturationOutDataTypeStr=Inherit: Same as second input  aMode=0
  Product : Product  Commented=on
  Product1 : Product  Commented=on
  S-R Flip Flops : Subsystem  Commented=on
  Saturation : Saturate  Commented=on  UpperLimit=22  LowerLimit=0
  Saturation1 : Saturate  Commented=on  UpperLimit=inf  LowerLimit=0
  Saturation2 : Saturate  Commented=on  UpperLimit=1  LowerLimit=-1
  Saturation3 : Saturate  Commented=on  UpperLimit=1  LowerLimit=-1
  Saturation4 : Saturate  UpperLimit=21  LowerLimit=0
  Saturation5 : Saturate  UpperLimit=0  LowerLimit=-inf
  Sliding Mode Controller : eeSlidingModeController/Sliding Mode Controller  Commented=on  h=0.2  up=10  lo=0  Ts=-1
      settings: SourceProductBaseCode=PS
  Slip Control : Subsystem  Commented=on
  Subsystem : Subsystem
  Subsystem1 : Subsystem
  Subtract : Sum  Commented=on  Inputs=+-
  Subtract1 : Sum  Commented=on  Inputs=+-
  Subtract2 : Sum  Commented=on  Inputs=+-
  Switch1 : Switch  Commented=on  Criteria=u2 > Threshold  Threshold=0.1  SaturateOnIntegerOverflow=off  InputSameDT=off
  TC_Activation_Logic : Stateflow chart  Commented=on  TreatAsAtomicUnit=on
  Terminator1 : Terminator  Commented=on
  Unit Delay : UnitDelay  Commented=on  SampleTime=-1  HasFrameUpgradeWarning=on
  Unit Delay1 : UnitDelay  Commented=on  SampleTime=-1  HasFrameUpgradeWarning=on
  Unit Delay2 : UnitDelay  Commented=on  SampleTime=-1  HasFrameUpgradeWarning=on
  Varying Transfer Function : cstblocks/Linear Parameter Varying/Varying Transfer Function  Commented=on  N=1
  Out Bus Element1 : Outport  PortName=TC_Torque  Element=Traction
  Out Bus Element2 : Outport  PortName=TC_Torque  Element=Regen
  wires:
  Constant9/1 -> Out Bus Element2/1
  Constant6/1 -> Out Bus Element1/1
  Slip Control/2(Tmin) -> Unit Delay1/1
  Slip Control/1(Tmax) -> Unit Delay2/1
  Subtract1/1 -> Terminator1/1
  Constant5/1 -> Less Than/2
  PID Controller/1 -> Subtract1/2
  Less Than/1 -> PID Controller/2
  Subtract/1 -> PID Controller/1, Less Than/1
  Low-Pass Filter (Discrete or Continuous)/1 -> Discrete Derivative/1
  Unit Delay/1 -> TC_Activation_Logic/2(t_actual)
  Constant17/1 -> TC_Activation_Logic/7(slip_ratio_target)
  Bus Element In5/1 -> TC_Activation_Logic/6(slip_ratio)  "slip_ratios"
  In Bus Element7/1 -> Unit Delay/1
  In Bus Element6/1 -> TC_Activation_Logic/3(rtd_flag)  "rtd_flag"
  In Bus Element5/1 -> TC_Activation_Logic/4(tc_flag)  "tc_flag"
  TC_Activation_Logic/1(t_max_pid) -> Saturation/1
  In Bus Element/1 -> TC_Activation_Logic/5(t_limit_positive)  "t_limit_positive"
  Constant/1 -> Divide/1
  Divide/1 -> Varying Transfer Function/2
  Constant1/1 -> Varying Transfer Function/4
  In Bus Element2/1 -> Load Transfer calculation/1(dynamics_data)
  Bus Element In2/1 -> Subtract/1  "slip_ratios"
  Bus Element In3/1 -> Switch1/2  "slip_ratios"
  In Bus Element3/1 -> Memory/1
  Memory/1 -> Subtract1/1
  Bus Element In7/1 -> Sliding Mode Controller/2
  Bus Element In4/1 -> Low-Pass Filter (Discrete or Continuous)/1  "slip_ratios"
  Constant3/1 -> Sliding Mode Controller/1
  Constant4/1 -> Switch1/3
  Discrete Derivative1/1 -> Product/1
  Discrete Derivative/1 -> Gain3/1
  Fuzzification/1(Fuzzy_Outputs) -> Product1/2
  Gain3/1 -> Saturation3/1
  Gain4/1 -> Saturation2/1
  In Bus Element4/1 -> Discrete Derivative1/1
  Load Transfer calculation/1(Fz [4x1]) -> Product/2
  Product/1 -> Gain4/1
  Saturation2/1 -> Fuzzification/2(mu_p_FL)  "mu_p"
  Saturation3/1 -> Fuzzification/1(kappa_p_FL)  "kappa_p"
  Sliding Mode Controller/1 -> Saturation1/1
  Constant2/1 -> Subtract/2
  Memory1/1 -> Product1/1
  In Bus Element9/1 -> IC/1
  Bus Element In6/1 -> IC1/1  "slip_ratios"
  Bus Element In8/1 -> Less Than1/1  "slip_ratios"
  Constant7/1 -> Less Than1/2
  Less Than2/1 -> S-R Flip Flops/2(Reset)
  Bus Element In9/1 -> Less Than2/1  "slip_ratios"
  Less Than1/1 -> S-R Flip Flops/1(Set)
  Constant8/1 -> Less Than2/2
  Subsystem/1(Output) -> Saturation4/1
  Subsystem1/1(Output) -> Saturation5/1
  In Bus Element1/1 -> IC2/1
  Bus Element In1/1 -> IC3/1  "slip_ratios"
  In Bus Element10/1 -> Slip Control/2(omega_wheels)
  In Bus Element11/1 -> Slip Control/3(throttle)
  In Bus Element12/1 -> Slip Control/4(brake)
  Constant10/1 -> Slip Control/5(RTD)
  Constant11/1 -> Slip Control/6(TCon)
  In Bus Element13/1 -> Slip Control/7(vx_car)
  In Bus Element14/1 -> Slip Control/8(vy_car)
  In Bus Element15/1 -> Slip Control/9(yaw_rate)
  In Bus Element16/1 -> Slip Control/10(delta)
  Constant13/1 -> Slip Control/12(T_limit_regen)
  Constant12/1 -> Slip Control/11(T_limit)
  In Bus Element8/1 -> Slip Control/1(T_actual)
  IC/1 -> Subsystem/1(dynamics_data)
  IC1/1 -> Subsystem/2(slip_ratio)
  IC2/1 -> Subsystem1/1(dynamics_data)
  IC3/1 -> Subsystem1/2(slip_ratio)
